simulink model "mod_no_lineal"  (R2013a)
settings: Solver=ode3  StartTime=0.0  StopTime=0.2  FixedStep=1e-4  RelTol=1e-3
PreLoadFcn:
  | initialization.m
InitFcn:
  | k_d = 1.18e-7
  | B_a = 1.23e-6
  | u_min = 1.25
  | k_t = 3.7e-3
  | k_v = 7.8e-3
  | L_a = 1.9e-3
  | I_G = 1.5e-5
  | R_a = 260e-3
  | m = 0.694
  | l_a = 0.18
  | I_x = 5.87e-3
  | I_y = 5.87e-3
  | I_z = 10.73e-3
  | gamma0 = -47.7e-3
  | gamma1=1.3e-3
  | gamma2=-1.44e-6
  | gamma3=5.19e-9
  | g=9.8
  | delta_t=1e-4
  | R=eye(3)
model workspace: external: MATLAB File /home/cesar/Documentos/Documentos/Matlab/TFG/TFG/initialization.m (data not in the file)
libraries: cstblocks x8
settings Model: Creator=root  LastModifiedBy=root

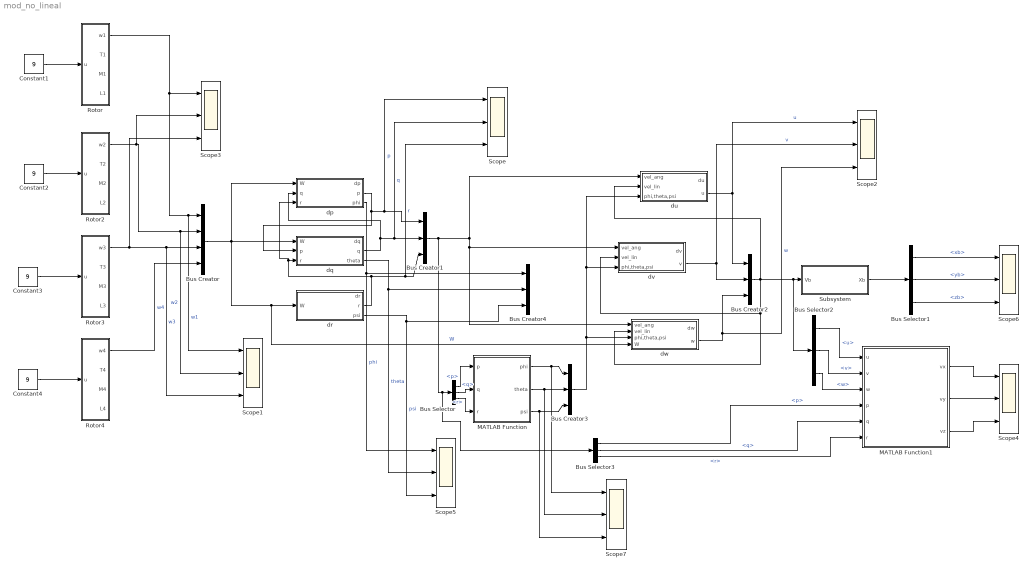
== system mod_no_lineal ==
  Bus Creator : BusCreator
  Bus Creator{1..4} (4 alike) : BusCreator  Inputs=3
  Bus Selector : BusSelector  OutputSignals=p,q,r
  Bus Selector1 : BusSelector  OutputSignals=xb,yb,zb
  Bus Selector2 : BusSelector  OutputSignals=u,v,w
  Bus Selector3 : BusSelector  OutputSignals=p,q,r
  Constant{1..4} (4 alike) : Constant  Value=9
  MATLAB Function : MATLAB Function  TreatAsAtomicUnit=on
  MATLAB Function1 : MATLAB Function  TreatAsAtomicUnit=on
  Rotor : Subsystem
  Rotor2 : Subsystem
  Rotor3 : Subsystem
  Rotor4 : Subsystem
  Scope{,1..7} (8 alike) : Scope  NumInputPorts=3
      Scope settings: YMin=-5~-5~-5  YMax=5~5~5
      Scope1 settings: YMin=-5~-5~-5  YMax=5~5~5  SaveName=ScopeData3
      Scope2 settings: YMin=-7~-1~-500  YMax=0~1~50
      Scope3 settings: YMin=-5~-5~-5  YMax=5~5~5  SaveName=ScopeData4
      Scope4 settings: YMin=-7~-1~-500  YMax=0~1~50  SaveName=ScopeData5
      Scope5 settings: YMin=-5~-5~-5  YMax=5~5~5  SaveName=ScopeData18
      Scope6 settings: YMin=-7~-1~-500  YMax=0~1~50  SaveName=ScopeData19
      Scope7 settings: YMin=-5~-5~-5  YMax=5~5~5  SaveName=ScopeData20
  Subsystem : Subsystem
  dp : Subsystem
  dq : Subsystem
  dr : Subsystem
  du : Subsystem
  dv : Subsystem
  dw : Subsystem
  wires:
  Constant1/1 -> Rotor/1(u)
  Rotor2/1(w2) -> Scope3/2, Scope1/2, Bus Creator/2  "w2"
  Rotor/1(w1) -> Scope3/1, Scope1/1, Bus Creator/1  "w1"
  Rotor3/1(w3) -> Scope3/3, Scope1/3, Bus Creator/3  "w3"
  Rotor4/1(w4) -> Bus Creator/4  "w4"
  Bus Creator/1 -> dp/1(W), dq/1(W), dw/4("W "), dr/1("W ")  "W"
  dp/2(p) -> Scope/1, Bus Creator1/1, dq/2("p ")  "p"
  dq/2(q) -> Scope/2, Bus Creator1/2, dp/2("q ")  "q"
  dr/2(r) -> Scope/3, Bus Creator1/3, dp/3(r), dq/3(r)  "r"
  Constant2/1 -> Rotor2/1(u)
  Constant3/1 -> Rotor3/1(u)
  Constant4/1 -> Rotor4/1(u)
  Bus Creator1/1 -> Bus Selector3/1, Bus Selector/1, dw/1(vel_ang), dv/1(vel_ang), du/1(vel_ang)
  dw/2(w) -> Scope2/3, Bus Creator2/3  "w"
  dv/2(v) -> Bus Creator2/2, Scope2/2  "v"
  du/2(u) -> Bus Creator2/1, Scope2/1  "u"
  Bus Creator2/1 -> Bus Selector2/1, Subsystem/1(Vb), du/2("vel_lin "), dw/2("vel_lin "), dv/2("vel_lin ")
  dp/3(phi) -> Bus Creator4/1, Scope5/1  "phi"
  dq/3(theta) -> Scope5/2, Bus Creator4/2  "theta"
  dr/3(psi) -> Bus Creator4/3, Scope5/3  "psi"
  Subsystem/1(Xb) -> Bus Selector1/1
  Bus Selector1/1 -> Scope6/1  "<xb>"
  Bus Selector1/2 -> Scope6/2  "<yb>"
  Bus Selector1/3 -> Scope6/3  "<zb>"
  Bus Selector/1 -> MATLAB Function/1(p)  "<p>"
  Bus Selector/2 -> MATLAB Function/2(q)  "<q>"
  Bus Selector/3 -> MATLAB Function/3(r)  "<r>"
  MATLAB Function/1(phi) -> Scope7/1, Bus Creator3/1
  MATLAB Function/2(theta) -> Scope7/2, Bus Creator3/2
  MATLAB Function/3(psi) -> Scope7/3, Bus Creator3/3
  Bus Creator3/1 -> du/3("phi,theta,psi "), dv/3("phi,theta,psi "), dw/3("phi,theta,psi ")
  Bus Selector2/1 -> MATLAB Function1/1(u)  "<u>"
  Bus Selector2/2 -> MATLAB Function1/2(v)  "<v>"
  Bus Selector2/3 -> MATLAB Function1/3(w)  "<w>"
  MATLAB Function1/1(vx) -> Scope4/1
  MATLAB Function1/2(vy) -> Scope4/2
  MATLAB Function1/3(vz) -> Scope4/3
  Bus Selector3/1 -> MATLAB Function1/4(p)  "<p>"
  Bus Selector3/2 -> MATLAB Function1/5(q)  "<q>"
  Bus Selector3/3 -> MATLAB Function1/6(r)  "<r>"

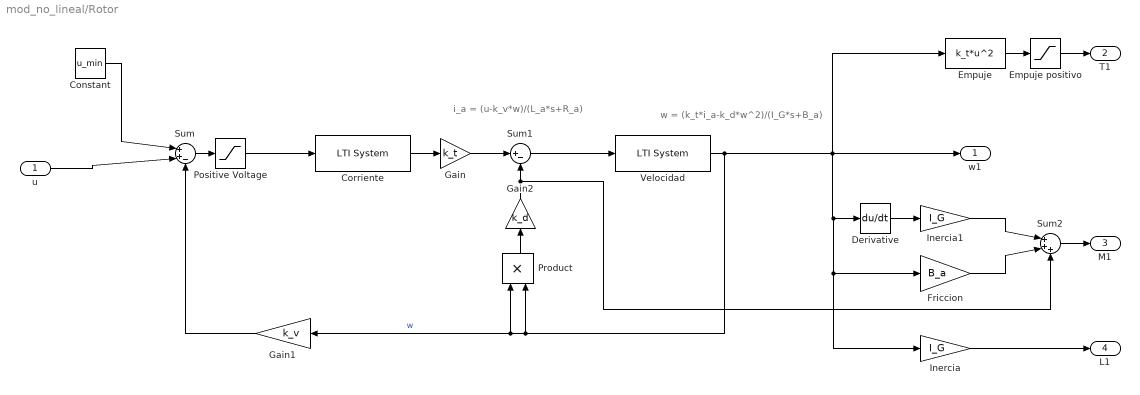
== system mod_no_lineal/Rotor ==
  note: w = (k_t*i_a-k_d*w^2)/(I_G*s+B_a)
  note: i_a = (u-k_v*w)/(L_a*s+R_a)
  u : Inport
  Constant : Constant  Value=u_min
  Corriente : cstblocks/LTI System  sys=tf(1,[L_a R_a])  IC=[]
  Derivative : Derivative
  Empuje : Fcn  Expr=k_t*u^2
  Empuje positivo : Saturate  UpperLimit=inf  LowerLimit=0
  Friccion : Gain  Gain=B_a
  Gain : Gain  Gain=k_t
  Gain1 : Gain  Gain=k_v
  Gain2 : Gain  Gain=k_d
  Inercia : Gain  Gain=I_G
  Inercia1 : Gain  Gain=I_G
  Positive Voltage : Saturate  UpperLimit=30  LowerLimit=0
  Product : Product
  Sum : Sum  Inputs=|++-
  Sum1 : Sum  Inputs=|+-
  Sum2 : Sum  Inputs=|+++
  Velocidad : cstblocks/LTI System  sys=tf(1,[I_G B_a])  IC=[]
  w1 : Outport
  T1 : Outport  Port=2
  M1 : Outport  Port=3
  L1 : Outport  Port=4
  wires:
  Gain2/1 -> Sum2/3, Sum1/2
  Gain1/1 -> Sum/3
  Velocidad/1 -> Inercia/1, Friccion/1, Derivative/1, Empuje/1, w1/1, Product/2, Product/1, Gain1/1  "w"
  u/1 -> Sum/2
  Corriente/1 -> Gain/1
  Sum1/1 -> Velocidad/1
  Product/1 -> Gain2/1
  Sum/1 -> Positive Voltage/1
  Constant/1 -> Sum/1
  Positive Voltage/1 -> Corriente/1
  Gain/1 -> Sum1/1
  Empuje/1 -> Empuje positivo/1
  Empuje positivo/1 -> T1/1
  Derivative/1 -> Inercia1/1
  Inercia1/1 -> Sum2/1
  Friccion/1 -> Sum2/2
  Sum2/1 -> M1/1
  Inercia/1 -> L1/1

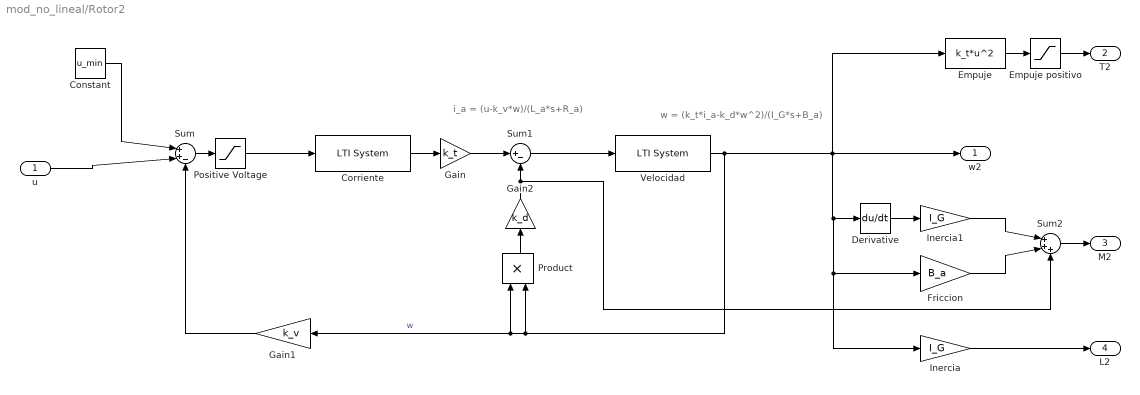
== system mod_no_lineal/Rotor2 ==
  note: i_a = (u-k_v*w)/(L_a*s+R_a)
  note: w = (k_t*i_a-k_d*w^2)/(I_G*s+B_a)
  u : Inport
  Constant : Constant  Value=u_min
  Corriente : cstblocks/LTI System  sys=tf(1,[L_a R_a])  IC=[]
  Derivative : Derivative
  Empuje : Fcn  Expr=k_t*u^2
  Empuje positivo : Saturate  UpperLimit=inf  LowerLimit=0
  Friccion : Gain  Gain=B_a
  Gain : Gain  Gain=k_t
  Gain1 : Gain  Gain=k_v
  Gain2 : Gain  Gain=k_d
  Inercia : Gain  Gain=I_G
  Inercia1 : Gain  Gain=I_G
  Positive Voltage : Saturate  UpperLimit=30  LowerLimit=0
  Product : Product
  Sum : Sum  Inputs=|++-
  Sum1 : Sum  Inputs=|+-
  Sum2 : Sum  Inputs=|+++
  Velocidad : cstblocks/LTI System  sys=tf(1,[I_G B_a])  IC=[]
  w2 : Outport
  T2 : Outport  Port=2
  M2 : Outport  Port=3
  L2 : Outport  Port=4
  wires:
  Inercia/1 -> L2/1
  Sum2/1 -> M2/1
  Friccion/1 -> Sum2/2
  Inercia1/1 -> Sum2/1
  Derivative/1 -> Inercia1/1
  Empuje positivo/1 -> T2/1
  Empuje/1 -> Empuje positivo/1
  Gain/1 -> Sum1/1
  Positive Voltage/1 -> Corriente/1
  Constant/1 -> Sum/1
  Sum/1 -> Positive Voltage/1
  Product/1 -> Gain2/1
  Sum1/1 -> Velocidad/1
  Corriente/1 -> Gain/1
  u/1 -> Sum/2
  Velocidad/1 -> Gain1/1, Product/1, Product/2, w2/1, Empuje/1, Derivative/1, Friccion/1, Inercia/1  "w"
  Gain1/1 -> Sum/3
  Gain2/1 -> Sum1/2, Sum2/3

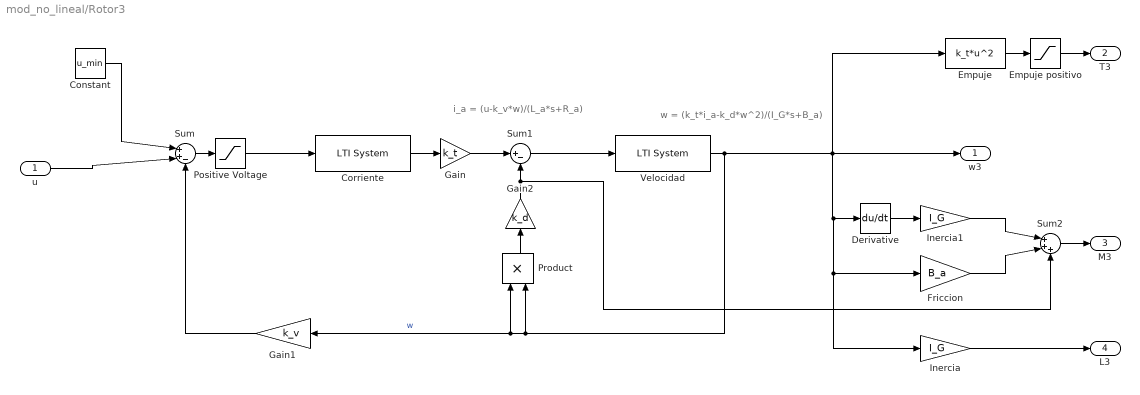
== system mod_no_lineal/Rotor3 ==
  note: w = (k_t*i_a-k_d*w^2)/(I_G*s+B_a)
  note: i_a = (u-k_v*w)/(L_a*s+R_a)
  u : Inport
  Constant : Constant  Value=u_min
  Corriente : cstblocks/LTI System  sys=tf(1,[L_a R_a])  IC=[]
  Derivative : Derivative
  Empuje : Fcn  Expr=k_t*u^2
  Empuje positivo : Saturate  UpperLimit=inf  LowerLimit=0
  Friccion : Gain  Gain=B_a
  Gain : Gain  Gain=k_t
  Gain1 : Gain  Gain=k_v
  Gain2 : Gain  Gain=k_d
  Inercia : Gain  Gain=I_G
  Inercia1 : Gain  Gain=I_G
  Positive Voltage : Saturate  UpperLimit=30  LowerLimit=0
  Product : Product
  Sum : Sum  Inputs=|++-
  Sum1 : Sum  Inputs=|+-
  Sum2 : Sum  Inputs=|+++
  Velocidad : cstblocks/LTI System  sys=tf(1,[I_G B_a])  IC=[]
  w3 : Outport
  T3 : Outport  Port=2
  M3 : Outport  Port=3
  L3 : Outport  Port=4
  wires:
  Gain2/1 -> Sum2/3, Sum1/2
  Gain1/1 -> Sum/3
  Velocidad/1 -> Inercia/1, Friccion/1, Derivative/1, Empuje/1, w3/1, Product/2, Product/1, Gain1/1  "w"
  u/1 -> Sum/2
  Corriente/1 -> Gain/1
  Sum1/1 -> Velocidad/1
  Product/1 -> Gain2/1
  Sum/1 -> Positive Voltage/1
  Constant/1 -> Sum/1
  Positive Voltage/1 -> Corriente/1
  Gain/1 -> Sum1/1
  Empuje/1 -> Empuje positivo/1
  Empuje positivo/1 -> T3/1
  Derivative/1 -> Inercia1/1
  Inercia1/1 -> Sum2/1
  Friccion/1 -> Sum2/2
  Sum2/1 -> M3/1
  Inercia/1 -> L3/1

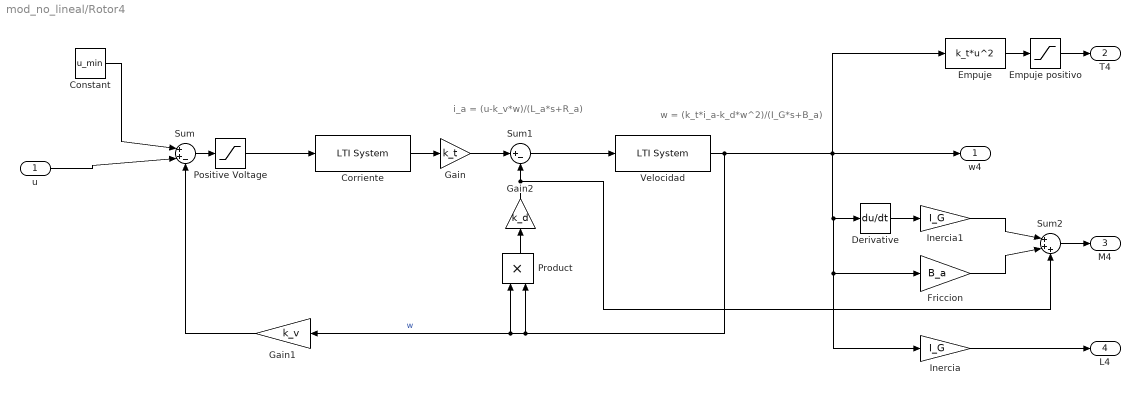
== system mod_no_lineal/Rotor4 ==
  note: i_a = (u-k_v*w)/(L_a*s+R_a)
  note: w = (k_t*i_a-k_d*w^2)/(I_G*s+B_a)
  u : Inport
  Constant : Constant  Value=u_min
  Corriente : cstblocks/LTI System  sys=tf(1,[L_a R_a])  IC=[]
  Derivative : Derivative
  Empuje : Fcn  Expr=k_t*u^2
  Empuje positivo : Saturate  UpperLimit=inf  LowerLimit=0
  Friccion : Gain  Gain=B_a
  Gain : Gain  Gain=k_t
  Gain1 : Gain  Gain=k_v
  Gain2 : Gain  Gain=k_d
  Inercia : Gain  Gain=I_G
  Inercia1 : Gain  Gain=I_G
  Positive Voltage : Saturate  UpperLimit=30  LowerLimit=0
  Product : Product
  Sum : Sum  Inputs=|++-
  Sum1 : Sum  Inputs=|+-
  Sum2 : Sum  Inputs=|+++
  Velocidad : cstblocks/LTI System  sys=tf(1,[I_G B_a])  IC=[]
  w4 : Outport
  T4 : Outport  Port=2
  M4 : Outport  Port=3
  L4 : Outport  Port=4
  wires:
  Inercia/1 -> L4/1
  Sum2/1 -> M4/1
  Friccion/1 -> Sum2/2
  Inercia1/1 -> Sum2/1
  Derivative/1 -> Inercia1/1
  Empuje positivo/1 -> T4/1
  Empuje/1 -> Empuje positivo/1
  Gain/1 -> Sum1/1
  Positive Voltage/1 -> Corriente/1
  Constant/1 -> Sum/1
  Sum/1 -> Positive Voltage/1
  Product/1 -> Gain2/1
  Sum1/1 -> Velocidad/1
  Corriente/1 -> Gain/1
  u/1 -> Sum/2
  Velocidad/1 -> Gain1/1, Product/1, Product/2, w4/1, Empuje/1, Derivative/1, Friccion/1, Inercia/1  "w"
  Gain1/1 -> Sum/3
  Gain2/1 -> Sum1/2, Sum2/3

== system mod_no_lineal/Subsystem ==
  Vb : Inport
  Bus Creator : BusCreator  Inputs=3
  Bus Selector : BusSelector  OutputSignals=u,v,w
  Integrator : Integrator
  Integrator1 : Integrator
  Integrator2 : Integrator
  Xb : Outport
  wires:
  Vb/1 -> Bus Selector/1
  Bus Selector/1 -> Integrator/1  "<u>"
  Bus Selector/2 -> Integrator1/1  "<v>"
  Bus Selector/3 -> Integrator2/1  "<w>"
  Integrator/1 -> Bus Creator/1  "xb"
  Integrator1/1 -> Bus Creator/2  "yb"
  Integrator2/1 -> Bus Creator/3  "zb"
  Bus Creator/1 -> Xb/1

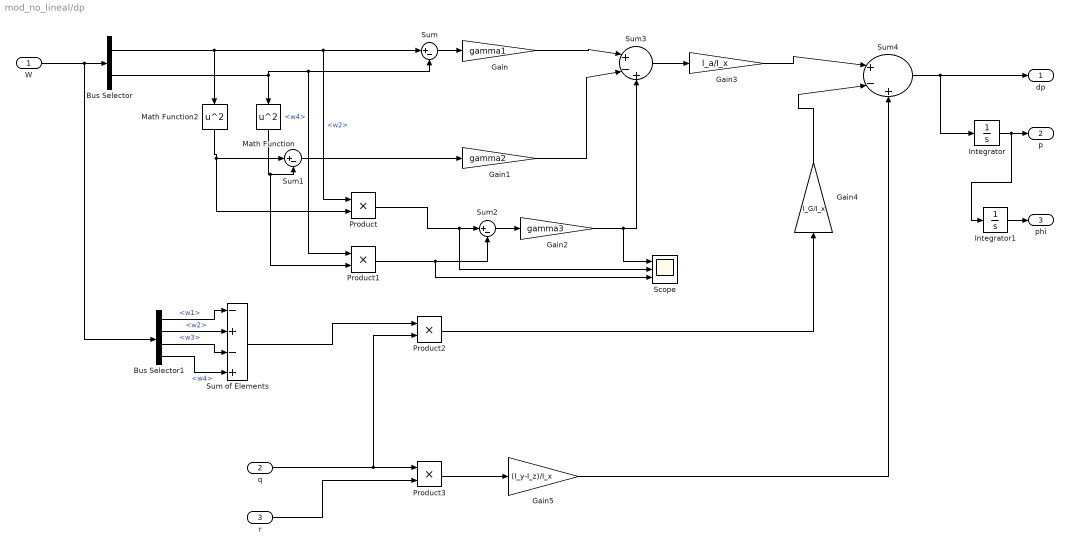
== system mod_no_lineal/dp ==
  W : Inport
  "q " : Inport  Port=2
  r : Inport  Port=3
  Bus Selector : BusSelector  OutputSignals=w2,w4
  Bus Selector1 : BusSelector  OutputSignals=w1,w2,w3,w4
  Gain : Gain  Gain=gamma1
  Gain1 : Gain  Gain=gamma2
  Gain2 : Gain  Gain=gamma3
  Gain3 : Gain  Gain=l_a/I_x
  Gain4 : Gain  Gain=I_G/I_x
  Gain5 : Gain  Gain=(I_y-I_z)/I_x
  Integrator : Integrator
  Integrator1 : Integrator
  Math Function : Math  Operator=square  SaturateOnIntegerOverflow=on
  Math Function2 : Math  Operator=square  SaturateOnIntegerOverflow=on
  Product{,1..3} (4 alike) : Product
  Scope : Scope  NumInputPorts=3
      settings: YMin=-5~-5~-5  YMax=5~5~5  SaveName=ScopeData2
  Sum : Sum  Inputs=|+-
  Sum of Elements : Sum  Inputs=-+-+
  Sum1 : Sum  Inputs=|+-
  Sum2 : Sum  Inputs=|+-
  Sum3 : Sum  Inputs=|+-+
  Sum4 : Sum  Inputs=|+-+
  dp : Outport
  p : Outport  Port=2
  phi : Outport  Port=3
  wires:
  W/1 -> Bus Selector1/1, Bus Selector/1
  Bus Selector/1 -> Product/1, Sum/1, Math Function2/1  "<w2>"
  Bus Selector/2 -> Product1/1, Sum/2, Math Function/1  "<w4>"
  Sum/1 -> Gain/1
  Gain/1 -> Sum3/1
  Math Function2/1 -> Product/2, Sum1/1
  Math Function/1 -> Product1/2, Sum1/2
  Sum1/1 -> Gain1/1
  Product/1 -> Scope/2, Sum2/1
  Product1/1 -> Scope/3, Sum2/2
  Sum2/1 -> Gain2/1
  Gain1/1 -> Sum3/2
  Gain2/1 -> Scope/1, Sum3/3
  Sum3/1 -> Gain3/1
  Gain3/1 -> Sum4/1
  Gain4/1 -> Sum4/2
  Bus Selector1/1 -> Sum of Elements/1  "<w1>"
  Bus Selector1/2 -> Sum of Elements/2  "<w2>"
  Bus Selector1/3 -> Sum of Elements/3  "<w3>"
  Bus Selector1/4 -> Sum of Elements/4  "<w4>"
  Sum of Elements/1 -> Product2/1
  "q "/1 -> Product2/2, Product3/1
  Product2/1 -> Gain4/1
  r/1 -> Product3/2
  Product3/1 -> Gain5/1
  Gain5/1 -> Sum4/3
  Integrator/1 -> Integrator1/1, p/1
  Integrator1/1 -> phi/1
  Sum4/1 -> Integrator/1, dp/1

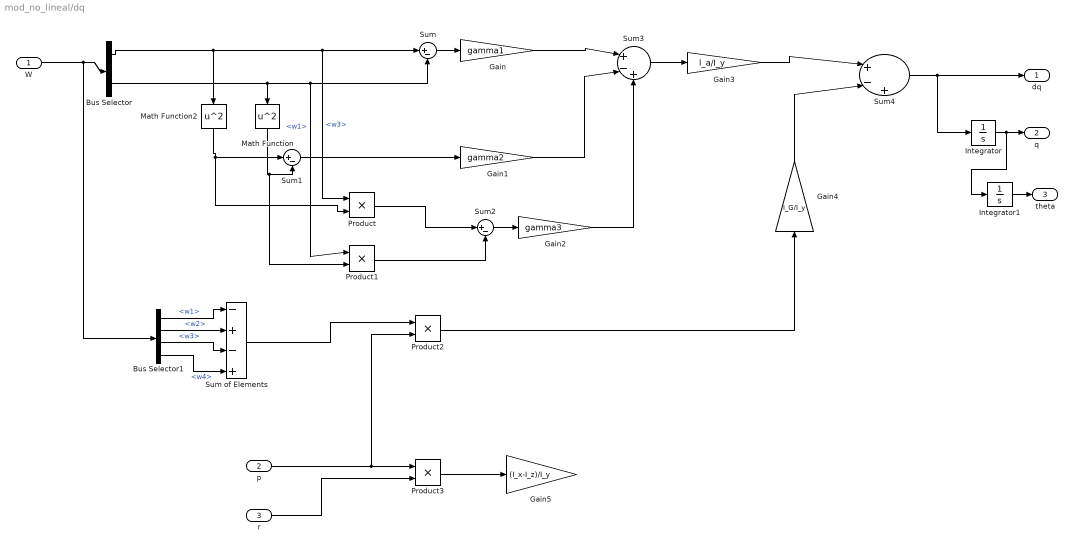
== system mod_no_lineal/dq ==
  W : Inport
  "p " : Inport  Port=2
  r : Inport  Port=3
  Bus Selector : BusSelector  OutputSignals=w3,w1
  Bus Selector1 : BusSelector  OutputSignals=w1,w2,w3,w4
  Gain : Gain  Gain=gamma1
  Gain1 : Gain  Gain=gamma2
  Gain2 : Gain  Gain=gamma3
  Gain3 : Gain  Gain=l_a/I_y
  Gain4 : Gain  Gain=I_G/I_y
  Gain5 : Gain  Gain=(I_x-I_z)/I_y
  Integrator : Integrator
  Integrator1 : Integrator
  Math Function : Math  Operator=square  SaturateOnIntegerOverflow=on
  Math Function2 : Math  Operator=square  SaturateOnIntegerOverflow=on
  Product{,1..3} (4 alike) : Product
  Sum : Sum  Inputs=|+-
  Sum of Elements : Sum  Inputs=-+-+
  Sum1 : Sum  Inputs=|+-
  Sum2 : Sum  Inputs=|+-
  Sum3 : Sum  Inputs=|+-+
  Sum4 : Sum  Inputs=|+-+
  dq : Outport
  q : Outport  Port=2
  theta : Outport  Port=3
  wires:
  W/1 -> Bus Selector1/1, Bus Selector/1
  Bus Selector/1 -> Product/1, Sum/1, Math Function2/1  "<w3>"
  Sum/1 -> Gain/1
  Gain/1 -> Sum3/1
  Math Function2/1 -> Product/2, Sum1/1
  Sum1/1 -> Gain1/1
  Product/1 -> Sum2/1
  Sum2/1 -> Gain2/1
  Gain1/1 -> Sum3/2
  Gain2/1 -> Sum3/3
  Sum3/1 -> Gain3/1
  Gain4/1 -> Sum4/2
  Bus Selector1/1 -> Sum of Elements/1  "<w1>"
  Bus Selector1/2 -> Sum of Elements/2  "<w2>"
  Bus Selector1/3 -> Sum of Elements/3  "<w3>"
  Bus Selector1/4 -> Sum of Elements/4  "<w4>"
  Sum of Elements/1 -> Product2/1
  "p "/1 -> Product2/2, Product3/1
  Product2/1 -> Gain4/1
  r/1 -> Product3/2
  Product3/1 -> Gain5/1
  Sum4/1 -> Integrator/1, dq/1
  Integrator/1 -> Integrator1/1, q/1
  Bus Selector/2 -> Product1/1, Sum/2, Math Function/1  "<w1>"
  Gain3/1 -> Sum4/1
  Math Function/1 -> Product1/2, Sum1/2
  Product1/1 -> Sum2/2
  Integrator1/1 -> theta/1

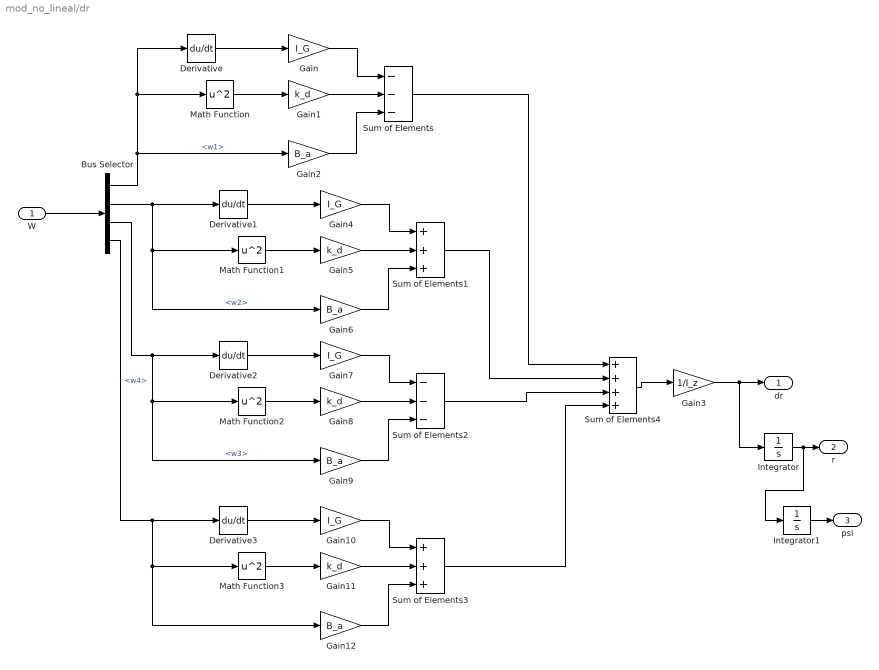
== system mod_no_lineal/dr ==
  "W " : Inport
  Bus Selector : BusSelector  OutputSignals=w1,w2,w3,w4
  Derivative{,1..3} (4 alike) : Derivative
  Gain{,4,7,10} (4 alike) : Gain  Gain=I_G
  Gain{1,5,8,11} (4 alike) : Gain  Gain=k_d
  Gain{2,6,9,12} (4 alike) : Gain  Gain=B_a
  Gain3 : Gain  Gain=1/I_z
  Integrator : Integrator
  Integrator1 : Integrator
  Math Function{,1..3} (4 alike) : Math  Operator=square  SaturateOnIntegerOverflow=on
  Sum of Elements : Sum  Inputs=---
  Sum of Elements1 : Sum  Inputs=+++
  Sum of Elements2 : Sum  Inputs=---
  Sum of Elements3 : Sum  Inputs=+++
  Sum of Elements4 : Sum  Inputs=++++
  dr : Outport
  r : Outport  Port=2
  psi : Outport  Port=3
  wires:
  "W "/1 -> Bus Selector/1
  Derivative/1 -> Gain/1
  Bus Selector/1 -> Math Function/1, Derivative/1, Gain2/1  "<w1>"
  Math Function/1 -> Gain1/1
  Gain/1 -> Sum of Elements/1
  Gain1/1 -> Sum of Elements/2
  Gain2/1 -> Sum of Elements/3
  Sum of Elements/1 -> Sum of Elements4/1
  Derivative1/1 -> Gain4/1
  Bus Selector/2 -> Gain6/1, Math Function1/1, Derivative1/1  "<w2>"
  Math Function1/1 -> Gain5/1
  Gain4/1 -> Sum of Elements1/1
  Gain5/1 -> Sum of Elements1/2
  Gain6/1 -> Sum of Elements1/3
  Sum of Elements1/1 -> Sum of Elements4/2
  Derivative2/1 -> Gain7/1
  Bus Selector/3 -> Derivative2/1, Math Function2/1, Gain9/1  "<w3>"
  Math Function2/1 -> Gain8/1
  Gain7/1 -> Sum of Elements2/1
  Gain8/1 -> Sum of Elements2/2
  Gain9/1 -> Sum of Elements2/3
  Sum of Elements2/1 -> Sum of Elements4/3
  Derivative3/1 -> Gain10/1
  Bus Selector/4 -> Gain12/1, Math Function3/1, Derivative3/1  "<w4>"
  Math Function3/1 -> Gain11/1
  Gain10/1 -> Sum of Elements3/1
  Gain11/1 -> Sum of Elements3/2
  Gain12/1 -> Sum of Elements3/3
  Sum of Elements3/1 -> Sum of Elements4/4
  Sum of Elements4/1 -> Gain3/1
  Integrator/1 -> Integrator1/1, r/1
  Gain3/1 -> Integrator/1, dr/1
  Integrator1/1 -> psi/1

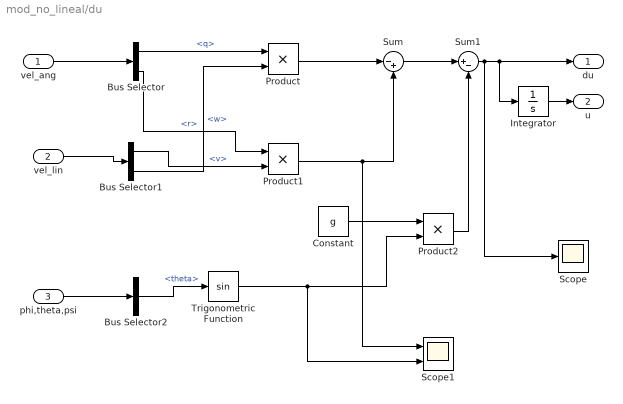
== system mod_no_lineal/du ==
  vel_ang : Inport
  "vel_lin " : Inport  Port=2
  "phi,theta,psi " : Inport  Port=3
  Bus Selector : BusSelector  OutputSignals=q,r
  Bus Selector1 : BusSelector  OutputSignals=v,w
  Bus Selector2 : BusSelector  OutputSignals=theta
  Constant : Constant  Value=g
  Integrator : Integrator
  Product : Product
  Product1 : Product
  Product2 : Product
  Scope : Scope
      settings: SaveName=ScopeData6
  Scope1 : Scope  NumInputPorts=2
      settings: YMin=-5~-5  YMax=5~5  SaveName=ScopeData7
  Sum : Sum  Inputs=|-+
  Sum1 : Sum  Inputs=|+-
  Trigonometric Function : Trigonometry
  du : Outport
  u : Outport  Port=2
  wires:
  vel_ang/1 -> Bus Selector/1
  "vel_lin "/1 -> Bus Selector1/1
  Bus Selector/1 -> Product/1  "<q>"
  Bus Selector1/2 -> Product/2  "<w>"
  Bus Selector/2 -> Product1/1  "<r>"
  Bus Selector1/1 -> Product1/2  "<v>"
  Product/1 -> Sum/1
  Product1/1 -> Scope1/1, Sum/2
  Sum/1 -> Sum1/1
  "phi,theta,psi "/1 -> Bus Selector2/1
  Constant/1 -> Product2/1
  Product2/1 -> Sum1/2
  Sum1/1 -> Scope/1, Integrator/1, du/1
  Integrator/1 -> u/1
  Bus Selector2/1 -> Trigonometric Function/1  "<theta>"
  Trigonometric Function/1 -> Scope1/2, Product2/2

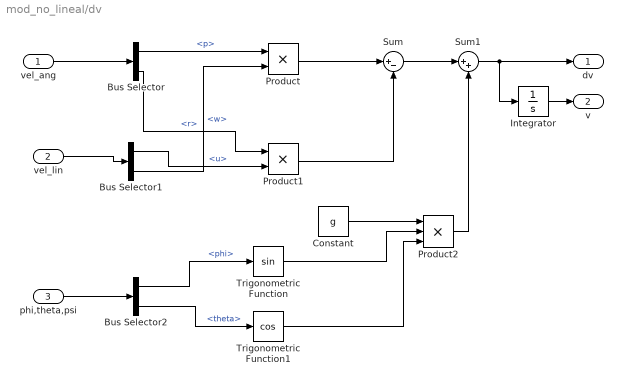
== system mod_no_lineal/dv ==
  vel_ang : Inport
  "vel_lin " : Inport  Port=2
  "phi,theta,psi " : Inport  Port=3
  Bus Selector : BusSelector  OutputSignals=p,r
  Bus Selector1 : BusSelector  OutputSignals=u,w
  Bus Selector2 : BusSelector  OutputSignals=phi,theta
  Constant : Constant  Value=g
  Integrator : Integrator
  Product : Product
  Product1 : Product
  Product2 : Product  Inputs=3
  Sum : Sum  Inputs=|+-
  Sum1 : Sum  Inputs=|++
  Trigonometric Function : Trigonometry
  Trigonometric Function1 : Trigonometry  Operator=cos
  dv : Outport
  v : Outport  Port=2
  wires:
  vel_ang/1 -> Bus Selector/1
  "vel_lin "/1 -> Bus Selector1/1
  Bus Selector/1 -> Product/1  "<p>"
  Bus Selector1/2 -> Product/2  "<w>"
  Bus Selector/2 -> Product1/1  "<r>"
  Bus Selector1/1 -> Product1/2  "<u>"
  Product/1 -> Sum/1
  Product1/1 -> Sum/2
  Sum/1 -> Sum1/1
  "phi,theta,psi "/1 -> Bus Selector2/1
  Constant/1 -> Product2/1
  Product2/1 -> Sum1/2
  Sum1/1 -> Integrator/1, dv/1
  Integrator/1 -> v/1
  Bus Selector2/1 -> Trigonometric Function/1  "<phi>"
  Bus Selector2/2 -> Trigonometric Function1/1  "<theta>"
  Trigonometric Function/1 -> Product2/2
  Trigonometric Function1/1 -> Product2/3

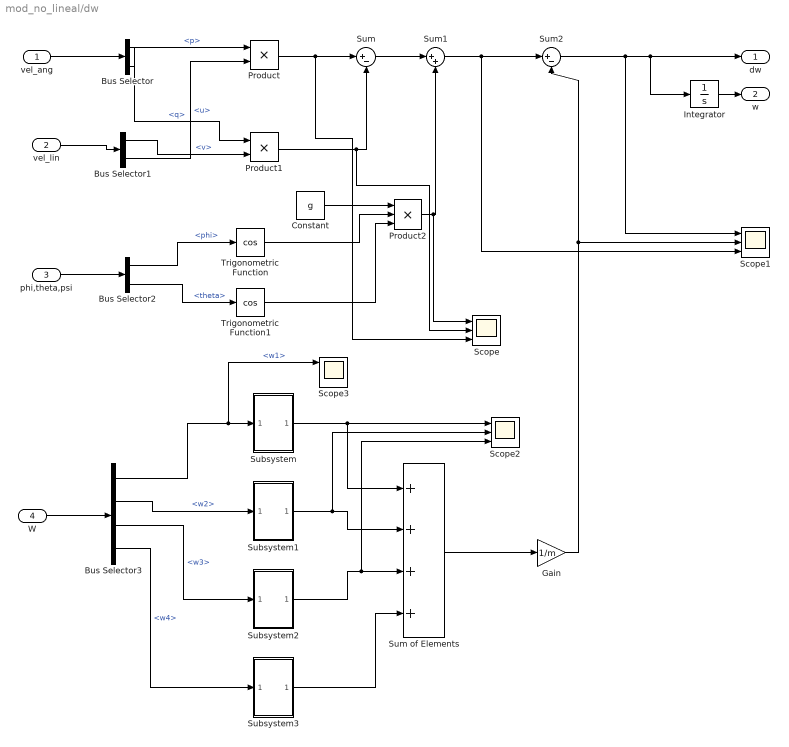
== system mod_no_lineal/dw ==
  vel_ang : Inport
  "vel_lin " : Inport  Port=2
  "phi,theta,psi " : Inport  Port=3
  "W " : Inport  Port=4
  Bus Selector : BusSelector  OutputSignals=q,p
  Bus Selector1 : BusSelector  OutputSignals=v,u
  Bus Selector2 : BusSelector  OutputSignals=phi,theta
  Bus Selector3 : BusSelector  OutputSignals=w1,w2,w3,w4
  Constant : Constant  Value=g
  Gain : Gain  Gain=1/m
  Integrator : Integrator
  Product : Product
  Product1 : Product
  Product2 : Product  Inputs=3
  Scope{,1..3} (4 alike) : Scope  NumInputPorts=3
      Scope settings: YMin=-5~-5~-5  YMax=5~5~5  SaveName=ScopeData8
      Scope1 settings: YMin=-800~-50~9.31  YMax=50~800~10.29  SaveName=ScopeData9
      Scope2 settings: YMin=-5~-5~-5  YMax=5~5~5  SaveName=ScopeData10
      Scope3 settings: YMin=-5~-5~-5  YMax=5~5~5  SaveName=ScopeData16
  Subsystem : Subsystem
  Subsystem1 : Subsystem
  Subsystem2 : Subsystem
  Subsystem3 : Subsystem
  Sum : Sum  Inputs=|+-
  Sum of Elements : Sum  Inputs=++++
  Sum1 : Sum  Inputs=|++
  Sum2 : Sum  Inputs=|+-
  Trigonometric Function : Trigonometry  Operator=cos
  Trigonometric Function1 : Trigonometry  Operator=cos
  dw : Outport
  w : Outport  Port=2
  wires:
  vel_ang/1 -> Bus Selector/1
  "vel_lin "/1 -> Bus Selector1/1
  Bus Selector/2 -> Product/1  "<p>"
  Bus Selector1/2 -> Product/2  "<u>"
  Bus Selector/1 -> Product1/1  "<q>"
  Bus Selector1/1 -> Product1/2  "<v>"
  Product/1 -> Scope/3, Sum/1
  Product1/1 -> Scope/2, Sum/2
  Sum/1 -> Sum1/1
  "phi,theta,psi "/1 -> Bus Selector2/1
  Constant/1 -> Product2/1
  Product2/1 -> Scope/1, Sum1/2
  Integrator/1 -> w/1
  Bus Selector2/1 -> Trigonometric Function/1  "<phi>"
  Bus Selector2/2 -> Trigonometric Function1/1  "<theta>"
  Trigonometric Function/1 -> Product2/2
  Trigonometric Function1/1 -> Product2/3
  Sum1/1 -> Scope1/3, Sum2/1
  "W "/1 -> Bus Selector3/1
  Bus Selector3/1 -> Scope3/1, Subsystem/1(In1)  "<w1>"
  Bus Selector3/2 -> Subsystem1/1(In1)  "<w2>"
  Bus Selector3/3 -> Subsystem2/1(In1)  "<w3>"
  Bus Selector3/4 -> Subsystem3/1(In1)  "<w4>"
  Subsystem/1(Out1) -> Sum of Elements/1, Scope2/1
  Subsystem1/1(Out1) -> Scope2/2, Sum of Elements/2
  Subsystem2/1(Out1) -> Scope2/3, Sum of Elements/3
  Subsystem3/1(Out1) -> Sum of Elements/4
  Sum of Elements/1 -> Gain/1
  Gain/1 -> Scope1/2, Sum2/2
  Sum2/1 -> Scope1/1, Integrator/1, dw/1

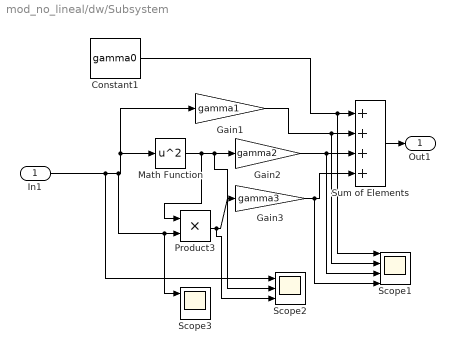
== system mod_no_lineal/dw/Subsystem ==
  In1 : Inport
  Constant1 : Constant  Value=gamma0
  Gain1 : Gain  Gain=gamma1
  Gain2 : Gain  Gain=gamma2
  Gain3 : Gain  Gain=gamma3
  Math Function : Math  Operator=square  SaturateOnIntegerOverflow=on
  Product3 : Product
  Scope1 : Scope  NumInputPorts=4
      settings: YMin=-5~-5~-5~-5  YMax=5~5~5~5  SaveName=ScopeData12
  Scope2 : Scope  NumInputPorts=3
      settings: YMin=-5~-5~-5  YMax=5~5~5  SaveName=ScopeData11
  Scope3 : Scope  NumInputPorts=3
      settings: YMin=-5~-5~-5  YMax=5~5~5  SaveName=ScopeData17
  Sum of Elements : Sum  Inputs=++++
  Out1 : Outport
  wires:
  In1/1 -> Scope2/1, Scope3/1, Product3/2, Math Function/1, Gain1/1
  Gain3/1 -> Scope1/4, Sum of Elements/4
  Sum of Elements/1 -> Out1/1
  Product3/1 -> Scope2/3, Gain3/1
  Constant1/1 -> Scope1/1, Sum of Elements/1
  Gain2/1 -> Scope1/3, Sum of Elements/3
  Math Function/1 -> Product3/1, Scope2/2, Gain2/1
  Gain1/1 -> Scope1/2, Sum of Elements/2

== system mod_no_lineal/dw/Subsystem1 ==
  In1 : Inport
  Constant1 : Constant  Value=gamma0
  Gain1 : Gain  Gain=gamma1
  Gain2 : Gain  Gain=gamma2
  Gain3 : Gain  Gain=gamma3
  Math Function : Math  Operator=square  SaturateOnIntegerOverflow=on
  Product3 : Product
  Scope1 : Scope  NumInputPorts=4
      settings: YMin=-5~-5~-5~-5  YMax=5~5~5~5  SaveName=ScopeData13
  Scope2 : Scope  NumInputPorts=4
      settings: YMin=-5~-5~-5~-5  YMax=5~5~5~5  SaveName=ScopeData14
  Scope3 : Scope  NumInputPorts=4
      settings: YMin=-5~-5~-5~-5  YMax=5~5~5~5  SaveName=ScopeData15
  Sum of Elements : Sum  Inputs=++++
  Out1 : Outport
  wires:
  Gain1/1 -> Scope3/1, Sum of Elements/2
  Math Function/1 -> Product3/1, Scope2/2, Gain2/1
  Gain2/1 -> Sum of Elements/3
  Constant1/1 -> Sum of Elements/1
  Product3/1 -> Scope2/3, Gain3/1
  Sum of Elements/1 -> Out1/1
  Gain3/1 -> Sum of Elements/4
  In1/1 -> Scope2/1, Gain1/1, Math Function/1, Product3/2
  ? -> Scope1/1

== system mod_no_lineal/dw/Subsystem2 ==
  In1 : Inport
  Constant1 : Constant  Value=gamma0
  Gain1 : Gain  Gain=gamma1
  Gain2 : Gain  Gain=gamma2
  Gain3 : Gain  Gain=gamma3
  Math Function : Math  Operator=square  SaturateOnIntegerOverflow=on
  Product3 : Product
  Sum of Elements : Sum  Inputs=++++
  Out1 : Outport
  wires:
  In1/1 -> Product3/2, Math Function/1, Gain1/1
  Gain3/1 -> Sum of Elements/4
  Sum of Elements/1 -> Out1/1
  Product3/1 -> Gain3/1
  Constant1/1 -> Sum of Elements/1
  Gain2/1 -> Sum of Elements/3
  Math Function/1 -> Product3/1, Gain2/1
  Gain1/1 -> Sum of Elements/2

== system mod_no_lineal/dw/Subsystem3 ==
  In1 : Inport
  Constant1 : Constant  Value=gamma0
  Gain1 : Gain  Gain=gamma1
  Gain2 : Gain  Gain=gamma2
  Gain3 : Gain  Gain=gamma3
  Math Function : Math  Operator=square  SaturateOnIntegerOverflow=on
  Product3 : Product
  Sum of Elements : Sum  Inputs=++++
  Out1 : Outport
  wires:
  Gain1/1 -> Sum of Elements/2
  Math Function/1 -> Product3/1, Gain2/1
  Gain2/1 -> Sum of Elements/3
  Constant1/1 -> Sum of Elements/1
  Product3/1 -> Gain3/1
  Sum of Elements/1 -> Out1/1
  Gain3/1 -> Sum of Elements/4
  In1/1 -> Gain1/1, Math Function/1, Product3/2

== matlab function mod_no_lineal/MATLAB Function1 ==
  data: u input; v input; w input; p input; q input; r input; vx output; vy output; vz output
function [vx,vy,vz] = transformmatrix(u,v,w,p,q,r)
%#codegen
%%
% Rotation matrix
persistent R

if isempty(R)
    R = eye(3)
end
vb = [u;v;w]

delta_t = 1e-4;
I = eye(3);
R_t = [0 -r*delta_t q*delta_t;r*delta_t 0 p*delta_t;-q*delta_t p*delta_t 0]
R = R*(eye(3)+ R_t)

v = R*vb

vx = v(1)
vy = v(2)
vz = v(3)

== matlab function mod_no_lineal/MATLAB Function ==
  data: p input; phi output; theta output; psi output; q input; r input
function [phi,theta,psi] = rotationmatrix(p,q,r)
%#codegen
%%
% Rotation matrix
persistent R

if isempty(R)
    R = eye(3)
end
delta_t = 1e-4;
I = eye(3);
R_t = [0 -r*delta_t q*delta_t;r*delta_t 0 p*delta_t;-q*delta_t p*delta_t 0]
R = R*(eye(3)+ R_t)

phi = atan(R(3,2)/R(3,3));
theta = -asin(R(3,1));
psi = atan(R(2,1)/R(1,1));

y = [phi theta psi];
